simulink model "gm_NewSignalGenerator"  (R2026a)
settings: Solver=VariableStepAuto  StopTime=5e-4
undefined symbols (not defined in the file or in its folder): ImTable, RealTable
libraries: hdlsllib x1, dsphdlxfrm2 x1
settings Model: Creator=adams  LastModifiedBy=adams
settings OptimizationCC: ConditionallyExecuteInputs=off
settings DebuggingCC: InheritedTsInSrcMsg=none

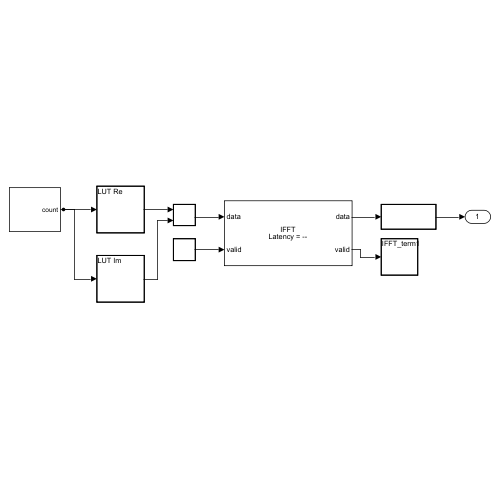
[thumbnail: Simulink's stored preview of the top-level diagram]
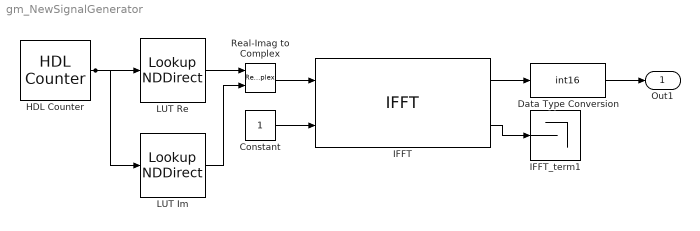
== system gm_NewSignalGenerator ==
  Constant : Constant  OutDataTypeStr=boolean
  Data Type Conversion : DataTypeConversion  OutDataTypeStr=int16  SaturateOnIntegerOverflow=off  RndMeth=Floor
  HDL Counter : hdlsllib/Sources/HDL Counter  CountType=Count limited  CountInit=0  CountStep=1  CountMax=511  CountFromType=Initial value  CountFrom=0  CountResetPort=off  CountLoadPort=off  CountEnbPort=off  CountDirPort=off  CountHitOutputPort=off  CountDataType=Unsigned  CountWordLen=9  CountFracLen=0  CountSampTime=2/614400000
  IFFT : dsphdlxfrm2/IFFT  Architecture=Streaming Radix 2^2  FFTLengthSource=Property  FFTLength=512  FFTLengthMax=1024  ComplexMultiplication=Use 4 multipliers and 2 adders  BitReversedOutput=off  BitReversedInput=off  Normalize=off  SimulateUsing=Code generation  RoundingMethod=Floor  ResetInputPort=off  StartOutputPort=off  EndOutputPort=off
  IFFT_term1 : Terminator
  LUT Im : LookupNDDirect  NumberOfTableDimensions=1  Table=ImTable  TableDataTypeStr=fixdt(1,32,20)
  LUT Re : LookupNDDirect  NumberOfTableDimensions=1  Table=RealTable  TableDataTypeStr=fixdt(1,32,20)
  Real-Imag to Complex : RealImagToComplex
  Out1 : Outport  SampleTime=3.25520833333333e-09
  wires:
  Constant/1 -> IFFT/2
  LUT Re/1 -> Real-Imag to Complex/1
  HDL Counter/1 -> LUT Re/1, LUT Im/1
  LUT Im/1 -> Real-Imag to Complex/2
  Real-Imag to Complex/1 -> IFFT/1
  IFFT/2 -> IFFT_term1/1
  IFFT/1 -> Data Type Conversion/1
  Data Type Conversion/1 -> Out1/1
